simulink model "Q2_b"  (R2022a)
settings: Solver=ode15s  StartTime=0.0  StopTime=20  RelTol=1e-3
settings Model: Creator=bhara  LastModifiedBy=manan
settings SolverCC: AlgebraicLoopSolver=TrustRegion
settings DebuggingCC: UnconnectedInputMsg=warning  UnconnectedOutputMsg=warning  UnconnectedLineMsg=warning  SFMachineParentedDataDiag=warning
settings RTWCC: DLArmComputeVersion=19.05

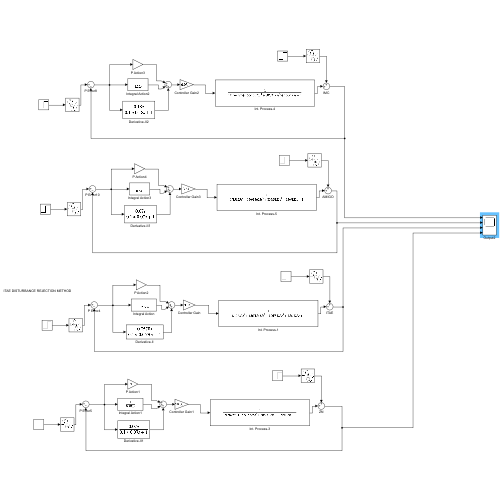
[thumbnail: Simulink's stored preview of the top-level diagram]
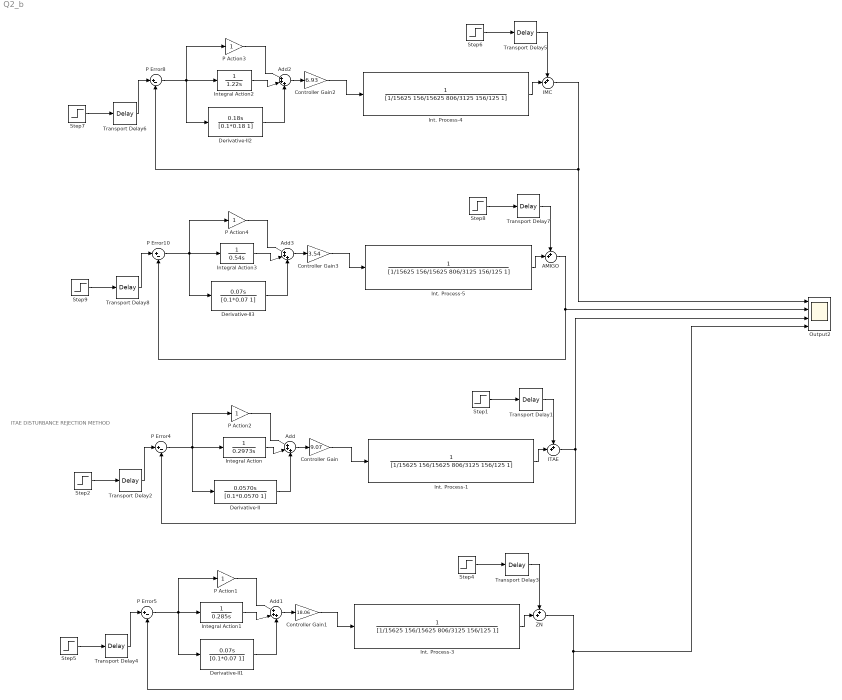
== system Q2_b ==
  note: ITAE DISTURBANCE REJECTION METHOD
  AMIGO : Sum  Inputs=++|
  Add{,1..3} (4 alike) : Sum  Inputs=|+++
  Controller Gain : Gain  Gain=9.07
  Controller Gain1 : Gain  Gain=18.06
  Controller Gain2 : Gain  Gain=6.93
  Controller Gain3 : Gain  Gain=3.54
  Derivative-II : TransferFcn  Numerator=[0.0570 0]  Denominator=[0.1*0.0570 1]
  Derivative-II1 : TransferFcn  Numerator=[0.07 0]  Denominator=[0.1*0.07 1]
  Derivative-II2 : TransferFcn  Numerator=[0.18 0]  Denominator=[0.1*0.18 1]
  Derivative-II3 : TransferFcn  Numerator=[0.07 0]  Denominator=[0.1*0.07 1]
  IMC : Sum  Inputs=++|
  ITAE : Sum  Inputs=++|
  Int. Process-{1,3..5} (4 alike) : TransferFcn  Denominator=[1/15625 156/15625 806/3125 156/125 1]
  Integral Action : TransferFcn  Denominator=[0.2973 0]
  Integral Action1 : TransferFcn  Denominator=[0.285 0]
  Integral Action2 : TransferFcn  Denominator=[1.22 0]
  Integral Action3 : TransferFcn  Denominator=[0.54 0]
  Output2 : Scope  NumInputPorts=4
  P Action{1..4} (4 alike) : Gain
  P Error{4..5,8,10} (4 alike) : Sum  Inputs=|+-
  Step{1..2,4..9} (8 alike) : Step  SampleTime=0
  Transport Delay{1,3,5,7} (4 alike) : TransportDelay  DelayTime=10
  Transport Delay{2,4,6,8} (4 alike) : TransportDelay
  ZN : Sum  Inputs=++|
  wires:
  Int. Process-1/1 -> ITAE/2
  Step1/1 -> Transport Delay1/1
  ITAE/1 -> P Error4/2, Output2/3
  Step2/1 -> Transport Delay2/1
  Controller Gain/1 -> Int. Process-1/1
  Transport Delay1/1 -> ITAE/1
  Add/1 -> Controller Gain/1
  Integral Action/1 -> Add/2
  P Action2/1 -> Add/1
  P Error4/1 -> P Action2/1, Integral Action/1, Derivative-II/1
  Derivative-II/1 -> Add/3
  Transport Delay2/1 -> P Error4/1
  P Error5/1 -> P Action1/1, Integral Action1/1, Derivative-II1/1
  Add1/1 -> Controller Gain1/1
  Integral Action1/1 -> Add1/2
  Derivative-II1/1 -> Add1/3
  P Action1/1 -> Add1/1
  Step5/1 -> Transport Delay4/1
  Step4/1 -> Transport Delay3/1
  Int. Process-3/1 -> ZN/2
  ZN/1 -> Output2/4, P Error5/2
  Transport Delay4/1 -> P Error5/1
  Transport Delay3/1 -> ZN/1
  Controller Gain1/1 -> Int. Process-3/1
  P Error8/1 -> P Action3/1, Integral Action2/1, Derivative-II2/1
  Add2/1 -> Controller Gain2/1
  Integral Action2/1 -> Add2/2
  Derivative-II2/1 -> Add2/3
  P Action3/1 -> Add2/1
  Step7/1 -> Transport Delay6/1
  Step6/1 -> Transport Delay5/1
  Int. Process-4/1 -> IMC/2
  IMC/1 -> Output2/1, P Error8/2
  Transport Delay6/1 -> P Error8/1
  Transport Delay5/1 -> IMC/1
  Controller Gain2/1 -> Int. Process-4/1
  P Error10/1 -> P Action4/1, Integral Action3/1, Derivative-II3/1
  Add3/1 -> Controller Gain3/1
  Integral Action3/1 -> Add3/2
  Derivative-II3/1 -> Add3/3
  P Action4/1 -> Add3/1
  Step9/1 -> Transport Delay8/1
  Step8/1 -> Transport Delay7/1
  Int. Process-5/1 -> AMIGO/2
  AMIGO/1 -> P Error10/2, Output2/2
  Transport Delay8/1 -> P Error10/1
  Transport Delay7/1 -> AMIGO/1
  Controller Gain3/1 -> Int. Process-5/1
